simulink model "DQGEN2"  (R2023b)
settings: Solver=ode23tb  StartTime=0.0  StopTime=1  FixedStep=Ts  RelTol=1e-5  EnableMultiTasking=on
values from neighbouring files (symbols this model uses):
  Cd = INVR*SYS.C*Ts    [DQGEN_calc.m]
  N = 2    [DQGEN_calc.m]
  Ts = 50e-6    (= 5e-05)    [DQGEN_calc.m]
  Ts_dqn = Ts    (= 5e-05)    [DQGEN_calc.m]
  Ws = 2*pi*f    (= 376.991118431)    [DQGEN_calc.m]
undefined symbols (not defined in the file or in its folder): ctrl1, Da, DiscIntNeverNeededParam, dtha, FA, Ha, InitVec, Ka, q0, rlc, SM, SMRD, SYS
libraries: spsabctodq0Lib x5, DQN_Lib x5, spsFirstOrderFilterLib x5, spsThreePhaseVIMeasurementLib x3, spsLoadFlowBusLib x2, spsMultimeterLib x2, spsThreePhaseSourceLib x1, spsdq0toabcLib x1, spsGroundLib x1, spsSynchronousMachinepuStandardLib x1, spsThreePhaseParallelRLCBranchLib x1, spsThreePhaseSeriesRLCBranchLib x1
(part 1 of 4)
settings Model: NumberOfSteps=10  PacingRate=0.005000  Creator=The MathWorks, Inc.  LastModifiedBy=rober
settings SolverCC: ZeroCrossControl=DisableAll  ZeroCrossAlgorithm=Adaptive  AlgebraicLoopSolver=TrustRegion
settings DataIOCC: SaveFormat=Array  SaveOutput=off  SaveTime=off  ReturnWorkspaceOutputs=off  TimeSaveName=t  SignalLoggingName=sigsOut
settings OptimizationCC: BlockReduction=off  BooleanDataType=off  ExpressionDepthLimit=2147483647  InitFltsAndDblsToZero=on  EfficientMapNaN2IntZero=off  LifeSpan=inf
settings DebuggingCC: UnderspecifiedInitializationDetection=Classic  MergeDetectMultiDrivingBlocksExec=none  CheckExecutionContextPreStartOutputMsg=on  SignalResolutionControl=TryResolveAllWithWarning  IgnoredZcDiagnostic=none  MultiTaskDSMMsg=warning  MultiTaskCondExecSysMsg=none  FcnCallInpInsideContextMsg=warning  StateNameClashWarn=warning  SFUnexpectedBacktrackingDiag=warning  SFNoUnconditionalDefaultTransitionDiag=warning  SFExecutionAtInitializationDiag=none  UnderSpecifiedDimensionMsg=warning  ArithmeticOperatorsInVariantConditions=warning
settings HardwareCC: ProdBitPerPointer=32  ProdBitPerSizeT=32  ProdBitPerPtrDiffT=32  ProdLargestAtomicFloat=None  ProdIntDivRoundTo=Undefined  ProdEndianess=Unspecified  ProdWordSize=32  ProdHWDeviceType=32-bit Generic  TargetBitPerPointer=64  TargetBitPerSizeT=64  TargetBitPerPtrDiffT=64  TargetLongLongMode=on  TargetIntDivRoundTo=Zero  TargetEndianess=LittleEndian  TargetWordSize=64  TargetHWDeviceType=MATLAB Host  ProdEqTarget=off
settings ModelReferenceCC: EnableRefExpFcnMdlSchedulingChecks=on  PropagateSignalLabelsOutOfModel=off
settings SFSimCC: SimUseLocalCustomCode=off  CustomCodeUndefinedFunction=UseInterfaceOnly
settings RTWCC: RTWUseLocalCustomCode=off  DLArmComputeVersion=19.05
settings CodeAppCC: StateflowObjectComments=on
settings GRTTargetCC: TargetLangStandard=C89/C90 (ANSI)  CombineOutputUpdateFcns=off  GRTInterface=on
settings ConfigComp: CovMetricSettings=dw  CovSaveCumulativeToWorkspaceVar=on  CovSaveSingleToWorkspaceVar=on  CovExternalEMLEnable=off  CovSFcnEnable=off
settings SimscapeCC: SimscapeNormalizeSystem=off

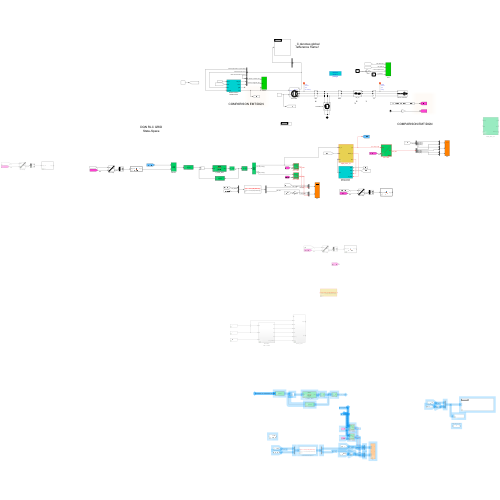
[thumbnail: Simulink's stored preview of the top-level diagram]
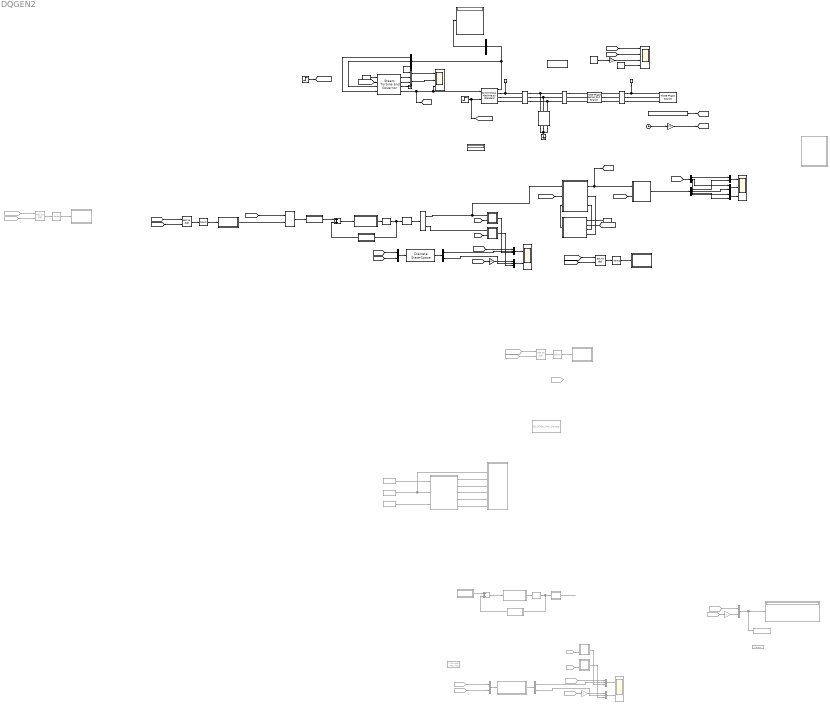
== system DQGEN2 ==
  note: DQN RLC GRID
      | State-Space
  note: 1
  note: 2
  note: 3
  note: 4
  note: COMPARISON EMT/DQN
  note: _C denotes global
      | refference frame!
  note: COMPARISON EMT/DQN
  500 kV 3333 MVA : spsThreePhaseSourceLib/Three-Phase Source  InternalConnection=Yg  VoltagePhases=off  Voltage=(24000)*1  PhaseAngle=0  Voltage_phases=[25e3 25e3 25e3]/sqrt(3)  PhaseAngles_phases=[0 -120 +120]  Frequency=60  NonIdealSource=off  SpecifyImpedance=on  Resistance=3.5  Inductance=0.1989  ShortCircuitLevel=3333e6  BaseVoltage=500e3  XRratio=21.43  BusType=swing  Pref=0  Qref=0  Prefabc=[10e3, 10e3, 10e3]  Qrefabc=[0, 0, 0]  Qmin=-Inf  Qmax=Inf
  Add1 : Sum
  Add2 : Sum  Commented=on
  B1 : spsThreePhaseVIMeasurementLib/Three-Phase V-I Measurement  VoltageMeasurement=phase-to-ground  SetLabelV=on  LabelV=Vabc_BSRC  Vpu=off  VpuLL=off  CurrentMeasurement=yes  SetLabelI=on  LabelI=Iabc_BSRC  Ipu=off  Pbase=100e6  Vbase=500e3  OutputType=Complex  PhasorSimulation=off  PSBequivalent=0
  B22 : spsThreePhaseVIMeasurementLib/Three-Phase V-I Measurement  VoltageMeasurement=phase-to-ground  SetLabelV=on  LabelV=Vabc_B22  Vpu=off  VpuLL=off  CurrentMeasurement=yes  SetLabelI=on  LabelI=Iabc_B222  Ipu=off  Pbase=555e6  Vbase=24e3  OutputType=Complex  PhasorSimulation=off  PSBequivalent=0
  B500 : spsThreePhaseVIMeasurementLib/Three-Phase V-I Measurement  VoltageMeasurement=phase-to-ground  SetLabelV=on  LabelV=Vabc_B500  Vpu=off  VpuLL=off  CurrentMeasurement=yes  SetLabelI=on  LabelI=Iabc_B500  Ipu=off  Pbase=100e6  Vbase=500e3  OutputType=Complex  PhasorSimulation=off  PSBequivalent=0
  Bus Selector1 : BusSelector  OutputSignals="Mechanical.Rotor angle deviation  d_theta (rad),Mechanical.Rotor speed  wm  (pu),Mechanical.Rotor speed deviation  dw (pu)"
  Bus Selector2 : BusSelector  OutputSignals="dq0 components.Stator voltage  vd (pu),dq0 components.Stator voltage  vq (pu),Load angle   delta  (deg)"  OutputAsBus=on
  Clock : Clock
  Constant1 : Constant
  Constant2 : Constant  Value=complex([ 0 (24e3)*sqrt(2/3); 0 0; 0 0])
  Constant3 : Constant  Commented=on  Value=SYS.A
  Constant5 : Constant
  Constant6 : Constant  Commented=on  Value=SYS.B
  Constant7 : Constant  Commented=on  Value=SYS.C
  DQN_Mac1_V1 : Subsystem  mask{HRM=N, NomParam=[ 555e6  24e3   60 ], reactVec=[1.81, 0.3, 0.23, 1.76, 0.65, 0.25, 0.15], timeConstVec=[ 1.3201, 0.0231, 0.3371, 0.0295 ], Rs=2.8544e-3, Mech=[ 0.8788  0 1 ], lfVec=[0.5396   -0.7334    1.0000    1.0315    0.4264], Ts=Ts, SW=on}
      mask prompts: HRM "Harmonic order:"; NomParam "Nominal power, line-to-line voltage, frequency [ Pn(VA)  Vn(Vrms)  fn(Hz) ]:"; reactVec "Reactances [ Xd  Xd'  Xd''  Xq  (Xq')  Xq''  Xl ] (pu):"; timeConstVec "[ Td'  Td''  (Tq')  Tq'' ] (s):"; Rs "Stator resistance Rs (pu):"; Mech "Inertia coefficient, friction factor, pole pairs [ H(s)  F(pu)  p()]:"; lfVec "Initial condition (phi(1x6), tho, dw) [1x8]:"; Ts "Integration timestep (s):"; SW "Method (dq - checked / abc - unchecked)"
      mask init:
      | SMRD = struct();
      | 
      |     SMRD.dwo = 0;
      | 
      |     SMRD.nState = numel(reactVec)-1;
      |     
      |     if(SMRD.nState>5)
      |         SMRD.RLinv   = zeros(6,6);
      |         SMRD.Linv    = zeros(6,6);
      |         SMRD.L       = zeros(6,6);
      |         SMRD.R       = zeros(6,6);
      |         W = zeros(6,6);
      |     else
      |         SMRD.RLinv   = zeros(5,5);
      |         SMRD.Linv    = zeros(5,5);
      |         SMRD.L       = zeros(5,5);
      |         SMRD.R       = zeros(5,5);
      |         W            = zeros(5,5);
      |     end
      | 
      |     SMRD.Rs      = Rs;
      | 
      |     SMRD.N       = 1;
      |     
      |     SMRD.H       = Mech(1);
      |     SMRD.F       = Mech(2);
      |     SMRD.p       = Mech(3);
      | 
      |     SMRD.Pn = NomParam(1);
      |     SMRD.Vn = NomParam(2);
      |     SMRD.fn = NomParam(3);
      |     
      |     
      |     Vb = SMRD.Vn*sqrt(2/3);
      |     Ib = sqrt(2/3)*SMRD.Pn/SMRD.Vn;
      |     
      |     
      |     Td_p    = timeConstVec(1);
      |     Td_pp   = timeConstVec(2);
      |     if(SMRD.nState>5)
      |         Tq_p    = timeConstVec(3);
      |         Tq_pp   = timeConstVec(4);
      |     else
      |         Tq_pp   = timeConstVec(3);
      |     end
      |     
      |     
      |     %Set the time constants in Lq(s)
      |     %See (eq. 7.2.14)
      |     
      |     wn=2*pi*SMRD.fn;
      |     SMRD.wn = wn;%Rated frequency in rad/sec
      |     %Implementation of the formulas in 
      |     
      |     % Xaq=1.165; %Mutual inductance
      |     % Ll=.188; %Stator leakage inductance
      |     
      |     %T5=0.0234;
      |     
      |     
      |     Xd      = reactVec(1);
      |     Xd_p    = reactVec(2);
      |     Xd_pp   = reactVec(3);
      |     Xq      = reactVec(4);
      | 
      | 
      |     if(SMRD.nState>5)
      |         Xq_p    = reactVec(5);
      |         Xq_pp   = reactVec(6);
      |         Xl      = reactVec(7);
      | 
      |         Tqo_p   = Tq_p * Xq/Xq_p;
      |         Tqo_pp  = Tq_pp * Xq_p/Xq_pp;
      |     else
      |         Xq_pp   = reactVec(5);
      |         Xl      = reactVec(6);
      |         Tqo_pp  = Tq_pp * Xq/Xq_pp;
      |     end
      | 
      | 
      |     Xad     = Xd-Xl; %Mutual inductance
      |     Xaq     = Xq-Xl; %Mutual inductance
      |     
      |     
      |     SMRD.Xd = Xd;
      |     SMRD.Xq = Xq;
      |     SMRD.Xl = Xl;
      |     SMRD.Xad = Xad;
      |     SMRD.Xaq = Xaq;
      |     
      |         
      |    
      |     LAM1 = sqrt(Xd^2*Xd_pp^2*(Td_p-Td_pp)^2+2*Td_p*Td_pp*Xd*Xd_p*Xd_pp*(Xd-2*Xd_p+Xd_pp)-2*Td_pp*Xd*Xd_p*Xd_pp*(Xd-Xd_p+Xd_pp)+Td_pp^2*Xd_pp^2*(Xd^2+Xd_pp^2));
      |     Tdo_p  = (Td_p*Xd*Xd_pp+LAM1+Td_pp*(Xd*Xd_p+Xd_p*Xd_pp-Xd*Xd_pp))/(2*Xd_p*Xd_pp);
      |     Tdo_pp = Xd*Td_p*Td_pp/(Xd_pp*Tdo_p);
      |     % 
      |     % Tqo_p   = Tq_p * Xq/Xq_p;
      |     % Tqo_pp  = Tq_pp * Xq_p/Xq_pp;
      | 
      | 
      |     % D-Axis
      |     a=SMRD.Xad*(Xd_p-SMRD.Xl)/(Xd-Xd_p);
      |     b=a*SMRD.Xad*(Xd_pp-SMRD.Xl)/(a*Xd+SMRD.Xl*SMRD.Xad-(a+SMRD.Xad)*Xd_pp);
      |     c=(b+a*SMRD.Xl*SMRD.Xad/(SMRD.Xl*SMRD.Xad+a*Xd))/Td_pp;
      |     
      |     T5 = b/c;
      | 
      |     if(1)
      |         a = Xad*(Xd_p-Xl)/(Xd-Xd_p);
      |         b = Xad*(Xd_pp-Xl)/(a*Xd+Xl*Xad-(a+Xad)*Xd_pp);
      |         c = (1/Td_pp)*(b-(a*Xl*Xad)/(Xl*Xad+a*Xd) );
      |         
      |         T11d = b/c;
      |     end
      | 
      |     
      |     if(1)
      |         %Set the time constants in Ld(s),sG(s)
      |         %See (eq. 7.2.4-7.2.5)
      |         T1 = Td_p; %T1=1.419; %Td'
      |         T2 = Td_pp; %T2=0.0669; %Td''
      |         T3 = Tdo_p; %T3=5.62; %Tdo'
      |         T4 = Tdo_pp; %T4=0.09; %Tdo''
      |         %T5 = T5; %T5=0.0234;
      |         Ld = Xd; %Ld= 1.104; %Synchronous inductance
      |         Ll = Xl; %Ll=0.198; %Stator leakage inductance
      |         Lad = Xad; %Lad=Ld-Ll; %Mutual inductance
      |         %Rated frequency in rad/sec
      |         %Implementation of the formulas in
      | 
      |         T5 = T11d;
      | 
      |         Ro=wn*Ld*(T3+T4-T1-T2);
      |         Ro=Lad*Lad/Ro;
      |         a=Ld*(T1+T2)-Ll*(T3+T4);a=a/Lad;
      |         b=Ld*T1*T2-Ll*T3*T4; b=b/Lad;
      |         c=(T3*T4-T1*T2)/(T3+T4-T1-T2);
      | 
      |         Lf1d=b-a*T5+T5*T5; %in p.u.
      |         Lf1d=Ro*Lf1d/(c-T5); %in p.u.
      |         Rfd=Ro*(Lf1d+Ro*(2*T5-a));
      |         Rfd=Rfd/(Lf1d+Ro*(T5+c-a));%in p.u.
      | 
      |         R1d=Ro*Rfd/(Rfd-Ro); %in p.u.
      |         %Inductances in p.u.
      |         L1d=R1d*T5; 
      |         L1d=L1d*wn;
      | 
      |         Lfd=Rfd*(a-T5-Lf1d/Ro); %in p.u.
      |         Lfd=Lfd*wn; 
      |         Lf1d=Lf1d*wn;
      | 
      |         SMRD.Lf1d = Lf1d;
      |         SMRD.Rfd = Rfd;
      |         SMRD.R1d = R1d;
      |         SMRD.L1d = L1d;
      |         SMRD.Lfd = Lfd;
      |     end
      | 
      | 
      |     %%%%%%%%%%%%%%%%%%%%%%%%% Q AXIS %%%%%%%%%%%%%%%%%%%%%%%%% Tqo′ Xq″ Xq SMRD.Xl 
      |     
      |     if(SMRD.nState>5)
      |         %conv(x,y)= polynomial multiplication
      |         N=conv([Tq_p 1],[Tq_pp 1]); 
      |         D=conv([Tqo_p 1],[Tqo_pp 1]);
      |         Nz=conv(N-D*SMRD.Xl/Xq,[Xaq/SMRD.wn 0]);
      |         Dz=D-N; Nz=Nz(1:3); Dz=Dz(1:2);
      |         Req=Nz(3)/Dz(2);
      |         Nz=Nz/Nz(3); Dz=Dz/Dz(2);
      |         %compute polynomial roots and sort them
      |         Tab=sort(abs(roots(Nz))); Tab=1./Tab;
      |         Tm=sort(abs(roots(Dz))); Tm=1/Tm(1);
      |         %Solve a system of two linear equa�tions
      |         x=[1 1;Tab(1) Tab(2)]\[1 ;Tm]/Req;
      |         %Results
      |         SMRD.R1q=1/x(1); 
      |         SMRD.L1q=SMRD.wn*SMRD.R1q*Tab(1); %in p.u.
      |         SMRD.R2q=1/x(2); 
      |         SMRD.L2q=SMRD.wn*SMRD.R2q*Tab(2); %in p.u.
      |     else
      |         N=conv([1],[Tq_pp 1]); 
      |         D=conv([1],[Tqo_pp 1]);
      |         Nz=conv(N-D*SMRD.Xl/Xq,[Xaq/SMRD.wn 0]);
      |         Dz=D-N; Nz=Nz(1:2); Dz=Dz(1:1);
      |         Req=Nz(2)/Dz(1);
      |         Nz=Nz/Nz(2); Dz=Dz/Dz(1);
      |         %compute polynomial roots and sort them
      |         Tab=sort(abs(roots(Nz))); Tab=1./Tab;
      |         Tm=1;
      |         %Solve a system of two linear equa�tions
      |         x=[1;Tab(1)]/Req;
      |         %Results
      |         SMRD.R1q=1/x(1); 
      |         SMRD.L1q=SMRD.wn*SMRD.R1q*Tab(1); %in p.u.
      |     end
      |     
      |     %%%%%%%%%%%%%%%%%%%%%%%%%%%%%%%%%%%%%%%%%%%%%%%%%%%%%%%%%%
      | 
      |     %%%%%%%%%%%%%%%%%%%%%%%%% R/L MAT %%%%%%%%%%%%%%%%%%%%%%%%%
      | 
      |     q_axis = 1;
      | 
      | 
      |     if(SMRD.nState>5) % D = 2,3,4 ; Q = 1,5,6
      | 
      |         if(q_axis)
      |             SMRD.L(2,2) = SMRD.Xd;  SMRD.L(2,3) = SMRD.Xad;                         SMRD.L(2,4) = SMRD.Xad; %D
      |             SMRD.L(3,2) = SMRD.Xad; SMRD.L(3,3) = SMRD.Xad + SMRD.Lf1d + SMRD.Lfd;  SMRD.L(3,4) = SMRD.Lf1d + SMRD.Xad; %D
      |             SMRD.L(4,2) = SMRD.Xad; SMRD.L(4,3) = SMRD.Xad + SMRD.Lf1d;             SMRD.L(4,4) = SMRD.Lf1d + SMRD.Xad + SMRD.L1d; %D
      | 
      |             SMRD.L(1,1) = SMRD.Xq;  SMRD.L(1,5) = SMRD.Xaq;                         SMRD.L(1,6) = SMRD.Xaq; %Q
      |             SMRD.L(5,1) = SMRD.Xaq; SMRD.L(5,5) = SMRD.Xaq + SMRD.L1q;              SMRD.L(5,6) = SMRD.Xaq; %Q
      |             SMRD.L(6,1) = SMRD.Xaq; SMRD.L(6,5) = SMRD.Xaq;                         SMRD.L(6,6) = SMRD.Xaq + SMRD.L2q; %Q
      | 
      | 
      |             SMRD.R(1,1) = Rs;
      |             SMRD.R(2,2) = Rs;
      |             SMRD.R(3,3) = SMRD.Rfd;
      |             SMRD.R(4,4) = SMRD.R1d;
      |             SMRD.R(5,5) = SMRD.R1q;
      |             SMRD.R(6,6) = SMRD.R2q;
      | 
      |         else
      |             SMRD.L(1,1) = SMRD.Xd;  SMRD.L(1,3) = SMRD.Xad;                         SMRD.L(1,5) = SMRD.Xad;
      |             SMRD.L(2,2) = SMRD.Xq;  SMRD.L(2,4) = SMRD.Xaq;                         SMRD.L(2,6) = SMRD.Xaq;
      |             SMRD.L(3,1) = SMRD.Xad; SMRD.L(3,3) = SMRD.Xad + SMRD.Lf1d + SMRD.Lfd;  SMRD.L(3,5) = SMRD.Lf1d + SMRD.Xad;
      |             SMRD.L(4,2) = SMRD.Xaq; SMRD.L(4,4) = SMRD.Xaq + SMRD.L1q;              SMRD.L(4,6) = SMRD.Xaq;
      |             SMRD.L(5,1) = SMRD.Xad; SMRD.L(5,3) = SMRD.Xad + SMRD.Lf1d;             SMRD.L(5,5) = SMRD.Lf1d + SMRD.Xad + SMRD.L1d;
      |             SMRD.L(6,2) = SMRD.Xaq; SMRD.L(6,4) = SMRD.Xaq;                         SMRD.L(6,6) = SMRD.Xaq  + SMRD.L2q;
      | 
      |             SMRD.R(1,1) = Rs;
      |             SMRD.R(2,2) = Rs;
      |             SMRD.R(3,3) = SMRD.Rfd;
      |             SMRD.R(4,4) = SMRD.R1q;
      |             SMRD.R(5,5) = SMRD.R1d;
      |             SMRD.R(6,6) = SMRD.R2q;
      |         end
      |     else
      | 
      |         if(q_axis)
      |             SMRD.L(2,2) = SMRD.Xd;  SMRD.L(2,3) = SMRD.Xad;                         SMRD.L(2,4) = SMRD.Xad;           %D
      |             SMRD.L(3,2) = SMRD.Xad; SMRD.L(3,3) = SMRD.Xad + SMRD.Lf1d + SMRD.Lfd;  SMRD.L(3,4) = SMRD.Lf1d + SMRD.Xad; %D
      |             SMRD.L(4,2) = SMRD.Xad; SMRD.L(4,3) = SMRD.Xad + SMRD.Lf1d;             SMRD.L(4,4) = SMRD.Lf1d + SMRD.Xad + SMRD.L1d;  %D
      |             
      |             SMRD.L(1,1) = SMRD.Xq;  SMRD.L(1,5) = SMRD.Xaq;              %Q
      |             SMRD.L(5,1) = SMRD.Xaq; SMRD.L(5,5) = SMRD.Xaq + SMRD.L1q;   %Q
      | 
      |             SMRD.R(1,1) = Rs;
      |             SMRD.R(2,2) = Rs;
      |             SMRD.R(3,3) = Rfd_R;
      |             SMRD.R(4,4) = R1d_R;
      |             SMRD.R(5,5) = SMRD.R1q;
      | 
      |         else
      |             SMRD.L(1,1) = SMRD.Xd; SMRD.L(1,3) = SMRD.Xad; SMRD.L(1,5) = SMRD.Xad;
      |             SMRD.L(2,2) = SMRD.Xq; SMRD.L(2,4) = SMRD.Xaq;
      |             SMRD.L(3,1) = SMRD.Xad; SMRD.L(3,3) = SMRD.Xad + SMRD.Lf1d + SMRD.L1d; SMRD.L(3,5) = SMRD.Lf1d + SMRD.Xad;
      |             SMRD.L(4,2) = SMRD.Xaq; SMRD.L(4,4) = SMRD.Xaq + SMRD.L1q; 
      |             SMRD.L(5,1) = SMRD.Xad; SMRD.L(5,3) = SMRD.Xad + SMRD.Lf1d; SMRD.L(5,5) = SMRD.Lf1d + SMRD.Xad + SMRD.Lfd;
      | 
      |             SMRD.R(1,1) = Rs;
      |             SMRD.R(2,2) = Rs;
      |             SMRD.R(3,3) = Rfd_R;
      |             SMRD.R(4,4) = SMRD.R1q;
      |             SMRD.R(5,5) = R1d_R;
      | 
      |         end
      |     end
      | 
      | 
      |    if(q_axis)
      |         W(2,1) = -1;
      |         W(1,2) = +1;
      |    else
      |         W(2,1) = +1;
      |         W(1,2) = -1;
      |    end
      |     
      |     %%%%%%%%%%%%%%%%%%%%%%%%%%%%% LF  %%%%%%%%%%%%%%%%%%%%%%%%%
      |     
      |     Pt = lfVec(1);
      |     Qt = lfVec(2);
      |     Vt = lfVec(3);
      |     Et = lfVec(4);
      |     At = lfVec(5);
      |     % if(numel(lfVec)>5) fac = lfVec(6); end
      |     
      |     phi = At;
      |     SMRD.phi = phi;
      | 
      |     SMRD.Vt = Vt*exp(1i*(phi));
      |     SMRD.It = (Pt-1i*Qt)/(Vt*exp(-1i*(phi)));
      |        
      |     %fi = sign(Qt)*acos(Pt/(Vt*It)); rad2deg(fi);
      |     fi = angle(SMRD.Vt)-angle(SMRD.It);
      |     SMRD.fi = fi;
      |     
      |     % del = (atan((Xq*It*cos(fi)-Rs*It*sin(fi))/(Vt+Rs*It*cos(fi)+Xq*It*sin(fi))));
      |     del = angle(SMRD.Vt+(SMRD.Rs+1i*SMRD.Xq)*SMRD.It)-(SMRD.phi);
      | 
      |     SMRD.del = del;
      | 
      |     SMRD.Vfnp = ((SMRD.Rfd*Vb/(Xad*wn))^2);
      |     
      |     v_dq = Vt*exp(1i*(pi/2-del)); %correct
      |     ed = real(v_dq);
      |     eq = imag(v_dq);
      |     efd = Et*SMRD.Vfnp;
      |     
      |    if(q_axis)
      |         v_vec = [eq; ed; efd; zeros(SMRD.nState-3,1)];
      |         i_vec = (v_vec'/(SMRD.R-SMRD.L*W))';
      |    else
      |         v_vec = [ed; eq; efd; zeros(SMRD.nState-3,1)];
      |         i_vec = (v_vec'/(SMRD.R-SMRD.L*W))';
      |    end
      | 
      |     %%%%%%%%%%%%%%%%%%%%%%%%%%%%%%%%%%%%%%%%%%%%%%%%%%%%%%%%%%
      |     
      |     SMRD.idq0 = i_vec;
      |     SMRD.phidq0 = SMRD.L*i_vec;
      |     
      |     SMRD.dwo = 0;
      | 
      |     SMRD.Linv = eye(SMRD.nState)/SMRD.L;
      |     
      |     if(1)
      |         SMRD.Linv2 = SMRD.Linv;
      |         SMRD.Linv2(3,4) = 0; SMRD.Linv2(4,3) = 0;
      |     end
      | 
      | 
      |     SMRD.RLinv = SMRD.R*SMRD.Linv;
      | 
      | 
      |     SMRD.Pb = 1;
      |     SMRD.Ib = Ib;
      |     SMRD.Vb = Vb;
      | 
      |     SMRD.IqdSign = [-1    -1     ones(1,SMRD.nState-2)];
      | 
      | 
      |     SMRD.Ts = Ts;
      |     SMRD.web = SMRD.wn;
      |     SMRD.v_dq = v_dq;
      | 
      |     tho = del+phi-pi/2;
      |     SMRD.tho = tho;
      settings: LibrarySourceBlock=|
      | spsSynchronousMachineModel/Continuous/Synchronous Machine
      | Continuous Model
  DQN_Mac_V1 : Subsystem  Commented=on  mask{HRM=N, NomParam=[ 555e6  24e3   60 ], reactVec=[1.81, 0.3, 0.23, 1.76, 0.65, 0.25, 0.15], timeConstVec=[ 1.3201, 0.0231, 0.3371, 0.0295 ], Rs=3.10E-03, Mech=[ 0.8788  0 1 ], lfVec=[0.9000   -0.0895    1.0000    1.8333    0.3334], Ts=Ts}
      mask prompts: HRM "Harmonic order:"; NomParam "Nominal power, line-to-line voltage, frequency [ Pn(VA)  Vn(Vrms)  fn(Hz) ]:"; reactVec "Reactances [ Xd  Xd'  Xd''  Xq  (Xq')  Xq''  Xl ] (pu):"; timeConstVec "[ Td'  Td''  (Tq')  Tq'' ] (s):"; Rs "Stator resistance Rs (pu):"; Mech "Inertia coefficient, friction factor, pole pairs [ H(s)  F(pu)  p()]:"; lfVec "Initial condition (phi(1x6), tho, dw) [1x8]:"; Ts "Integration timestep (s):"
      mask init:
      | SMRD = struct();
      | 
      |     SMRD.dwo = 0;
      | 
      |     SMRD.nState = numel(reactVec)-1;
      |     
      |     if(SMRD.nState>5)
      |         SMRD.RLinv   = zeros(6,6);
      |         SMRD.Linv    = zeros(6,6);
      |         SMRD.L       = zeros(6,6);
      |         SMRD.R       = zeros(6,6);
      |         W = zeros(6,6);
      |     else
      |         SMRD.RLinv   = zeros(5,5);
      |         SMRD.Linv    = zeros(5,5);
      |         SMRD.L       = zeros(5,5);
      |         SMRD.R       = zeros(5,5);
      |         W            = zeros(5,5);
      |     end
      | 
      |     SMRD.Rs      = Rs;
      | 
      |     SMRD.N       = 1;
      |     
      |     SMRD.H       = Mech(1);
      |     SMRD.F       = Mech(2);
      |     SMRD.p       = Mech(3);
      | 
      |     SMRD.Pn = NomParam(1);
      |     SMRD.Vn = NomParam(2);
      |     SMRD.fn = NomParam(3);
      |     
      |     
      |     Vb = SMRD.Vn*sqrt(2/3);
      |     Ib = sqrt(2/3)*SMRD.Pn/SMRD.Vn;
      |     
      |     
      |     Td_p    = timeConstVec(1);
      |     Td_pp   = timeConstVec(2);
      |     if(SMRD.nState>5)
      |         Tq_p    = timeConstVec(3);
      |         Tq_pp   = timeConstVec(4);
      |     else
      |         Tq_pp   = timeConstVec(3);
      |     end
      |     
      |     
      |     %Set the time constants in Lq(s)
      |     %See (eq. 7.2.14)
      |     
      |     wn=2*pi*SMRD.fn;
      |     SMRD.wn = wn;%Rated frequency in rad/sec
      |     %Implementation of the formulas in 
      |     
      |     % Xaq=1.165; %Mutual inductance
      |     % Ll=.188; %Stator leakage inductance
      |     
      |     %T5=0.0234;
      |     
      |     
      |     Xd      = reactVec(1);
      |     Xd_p    = reactVec(2);
      |     Xd_pp   = reactVec(3);
      |     Xq      = reactVec(4);
      | 
      | 
      |     if(SMRD.nState>5)
      |         Xq_p    = reactVec(5);
      |         Xq_pp   = reactVec(6);
      |         Xl      = reactVec(7);
      | 
      |         Tqo_p   = Tq_p * Xq/Xq_p;
      |         Tqo_pp  = Tq_pp * Xq_p/Xq_pp;
      |     else
      |         Xq_pp   = reactVec(5);
      |         Xl      = reactVec(6);
      |         Tqo_pp  = Tq_pp * Xq/Xq_pp;
      |     end
      | 
      | 
      |     Xad     = Xd-Xl; %Mutual inductance
      |     Xaq     = Xq-Xl; %Mutual inductance
      |     
      |     
      |     SMRD.Xd = Xd;
      |     SMRD.Xq = Xq;
      |     SMRD.Xl = Xl;
      |     SMRD.Xad = Xad;
      |     SMRD.Xaq = Xaq;
      |     
      |         
      |    
      |     LAM1 = sqrt(Xd^2*Xd_pp^2*(Td_p-Td_pp)^2+2*Td_p*Td_pp*Xd*Xd_p*Xd_pp*(Xd-2*Xd_p+Xd_pp)-2*Td_pp*Xd*Xd_p*Xd_pp*(Xd-Xd_p+Xd_pp)+Td_pp^2*Xd_pp^2*(Xd^2+Xd_pp^2));
      |     Tdo_p  = (Td_p*Xd*Xd_pp+LAM1+Td_pp*(Xd*Xd_p+Xd_p*Xd_pp-Xd*Xd_pp))/(2*Xd_p*Xd_pp);
      |     Tdo_pp = Xd*Td_p*Td_pp/(Xd_pp*Tdo_p);
      |     % 
      |     % Tqo_p   = Tq_p * Xq/Xq_p;
      |     % Tqo_pp  = Tq_pp * Xq_p/Xq_pp;
      |     
      |    
      |     %%%%%%%%%%%%%%%%%%%%%%
      |         
      |     a=SMRD.Xad*(Xd_p-SMRD.Xl)/(Xd-Xd_p);
      |     b=a*SMRD.Xad*(Xd_pp-SMRD.Xl)/(a*Xd+SMRD.Xl*SMRD.Xad-(a+SMRD.Xad)*Xd_pp);
      |     c=(b+a*SMRD.Xl*SMRD.Xad/(SMRD.Xl*SMRD.Xad+a*Xd))/Td_pp;
      |     
      |     T5 = b/c;
      |     
      |     %%%%%%%%%%%%%%%%%%%%%%%%% D AXIS %%%%%%%%%%%%%%%%%%%%%%%%%
      |     
      |     SMRD.Ro=SMRD.wn*Xd*(Tdo_p+Tdo_pp-Td_p-Td_pp);
      |     SMRD.Ro=SMRD.Xad*SMRD.Xad/SMRD.Ro;
      |     
      |     
      |     a=Xd*(Td_p+Td_pp)-SMRD.Xl*(Tdo_p+Tdo_pp);a=a/SMRD.Xad;
      |     b=Xd*Td_p*Td_pp-SMRD.Xl*Tdo_p*Tdo_pp; b=b/SMRD.Xad;
      |     c=(Tdo_p*Tdo_pp-Td_p*Td_pp)/(Tdo_p+Tdo_pp-Td_p-Td_pp);
      |     
      |     % T5=0.0234;
      |     
      |     SMRD.Lf1d=b-a*T5+T5*T5; %in p.u.
      |     SMRD.Lf1d=SMRD.Ro*SMRD.Lf1d/(c-T5); %in p.u.
      |     SMRD.Rfd=SMRD.Ro*(SMRD.Lf1d+SMRD.Ro*(2*T5-a)); 
      |     SMRD.Rfd=SMRD.Rfd/(SMRD.Lf1d+SMRD.Ro*(T5+c-a));%in p.u.
      |     SMRD.Lfd=SMRD.Rfd*(a-T5-SMRD.Lf1d/SMRD.Ro); %in p.u.
      |     SMRD.R1d=SMRD.Ro*SMRD.Rfd/(SMRD.Rfd-SMRD.Ro); %in p.u. 
      |     %Inductances in p.u.
      |     SMRD.L1d=SMRD.R1d*T5; SMRD.L1d=SMRD.L1d*SMRD.wn; 
      |     SMRD.Lfd=SMRD.Lfd*SMRD.wn; SMRD.Lf1d=SMRD.Lf1d*SMRD.wn;
      |     
      |     %%%%%%%%%%%%%%%%%%%%%%%%%%%%%%%%%%%%%%%%%%%%%%%%%%%%%%%%%%
      |     
      |     %%%%%%%%%%%%%%%%%%%%%%%%% Q AXIS %%%%%%%%%%%%%%%%%%%%%%%%% Tqo′ Xq″ Xq SMRD.Xl 
      |     
      |     if(SMRD.nState>5)
      |         %conv(x,y)= polynomial multiplication
      |         N=conv([Tq_p 1],[Tq_pp 1]); 
      |         D=conv([Tqo_p 1],[Tqo_pp 1]);
      |         Nz=conv(N-D*SMRD.Xl/Xq,[Xaq/SMRD.wn 0]);
      |         Dz=D-N; Nz=Nz(1:3); Dz=Dz(1:2);
      |         Req=Nz(3)/Dz(2);
      |         Nz=Nz/Nz(3); Dz=Dz/Dz(2);
      |         %compute polynomial roots and sort them
      |         Tab=sort(abs(roots(Nz))); Tab=1./Tab;
      |         Tm=sort(abs(roots(Dz))); Tm=1/Tm(1);
      |         %Solve a system of two linear equa�tions
      |         x=[1 1;Tab(1) Tab(2)]\[1 ;Tm]/Req;
      |         %Results
      |         SMRD.R1q=1/x(1); 
      |         SMRD.L1q=SMRD.wn*SMRD.R1q*Tab(1); %in p.u.
      |         SMRD.R2q=1/x(2); 
      |         SMRD.L2q=SMRD.wn*SMRD.R2q*Tab(2); %in p.u.
      |     else
      |         N=conv([1],[Tq_pp 1]); 
      |         D=conv([1],[Tqo_pp 1]);
      |         Nz=conv(N-D*SMRD.Xl/Xq,[Xaq/SMRD.wn 0]);
      |         Dz=D-N; Nz=Nz(1:2); Dz=Dz(1:1);
      |         Req=Nz(2)/Dz(1);
      |         Nz=Nz/Nz(2); Dz=Dz/Dz(1);
      |         %compute polynomial roots and sort them
      |         Tab=sort(abs(roots(Nz))); Tab=1./Tab;
      |         Tm=1;
      |         %Solve a system of two linear equa�tions
      |         x=[1;Tab(1)]/Req;
      |         %Results
      |         SMRD.R1q=1/x(1); 
      |         SMRD.L1q=SMRD.wn*SMRD.R1q*Tab(1); %in p.u.
      |     end
      |     
      |     %%%%%%%%%%%%%%%%%%%%%%%%%%%%%%%%%%%%%%%%%%%%%%%%%%%%%%%%%%
      |     
      |     
      |     if(1)
      |         T11d = T5;
      |         
      |         K1 = (Tdo_p+Tdo_pp-Td_p-Td_pp)*(Tdo_p*Tdo_pp*(Td_p+Td_pp)-Td_p*Td_pp*(Tdo_p+Tdo_pp))-(Tdo_p*Tdo_pp-Td_p*Td_pp)^2;    
      |         
      |         
      |         %K2 = Rfd*K1*Ld/(Lad^2);
      |         K2 = (Tdo_p*Tdo_pp*(Td_p+Td_pp)-Td_p*Td_pp*(Tdo_p+Tdo_pp)+T11d^2*(Tdo_p+Tdo_pp-Td_p-Td_pp)-2*T11d*(Tdo_p*Tdo_pp-Td_p*Td_pp))/SMRD.wn;
      |         K3 = Tdo_p*Tdo_pp-T11d*(Tdo_p+Tdo_pp-T11d);
      |         K4 = Tdo_p*Tdo_pp-Td_p*Td_pp-T11d*(Tdo_p+Tdo_pp-Td_p-Td_pp);
      |         K5 = Tdo_p*Tdo_pp*(Td_p+Td_pp)-Td_p*Td_pp*(Tdo_p+Tdo_pp)-T11d*(Tdo_p*Tdo_pp-Td_p*Td_pp);
      |         
      |         Rfd_R = Xad^2*K2/(Xd*K1);
      |         
      |         Lf1d_R = (Xad^2*K3/(Xd*K4)-Xad)*wn; %Lf1d
      |         Lfd_R = Rfd_R*K5/K4*wn; %Lfd
      |         R1d_R = Rfd_R*K1/K4^2;
      |         L1d_R = Rfd_R*T5*wn;
      |         
      |         SMRD.Rfd_R  = Rfd_R;
      |         SMRD.Lf1d_R = Lf1d_R;
      |         SMRD.Lfd_R = Lfd_R;
      |         SMRD.R1d_R = R1d_R;
      |         SMRD.L1d_R = L1d_R;
      |     end
      |     
      | 
      |     %%%%%%%%%%%%%%%%%%%%%%%%% R/L MAT %%%%%%%%%%%%%%%%%%%%%%%%%
      | 
      |     Ro=Xad*Xad/(wn*Xd*(Tdo_p+Tdo_pp-Td_p-Td_pp));
      | 
      |     if(SMRD.nState>5)
      |         SMRD.L(1,1) = SMRD.Xd; SMRD.L(1,3) = SMRD.Xad; SMRD.L(1,5) = SMRD.Xad;
      |         SMRD.L(2,2) = SMRD.Xq; SMRD.L(2,4) = SMRD.Xaq; SMRD.L(2,6) = SMRD.Xaq;
      |         SMRD.L(3,1) = SMRD.Xad; SMRD.L(3,3) = SMRD.Xad + SMRD.Lf1d + SMRD.L1d; SMRD.L(3,5) = SMRD.Lf1d + SMRD.Xad;
      |         SMRD.L(4,2) = SMRD.Xaq; SMRD.L(4,4) = SMRD.Xaq + SMRD.L1q; SMRD.L(4,6) = SMRD.Xaq;
      |         SMRD.L(5,1) = SMRD.Xad; SMRD.L(5,3) = SMRD.Xad + SMRD.Lf1d; SMRD.L(5,5) = SMRD.Lf1d + SMRD.Xad + SMRD.Lfd;
      |         SMRD.L(6,2) = SMRD.Xaq; SMRD.L(6,4) = SMRD.Xaq; SMRD.L(6,6) = SMRD.Xaq + SMRD.L2q;
      |     else
      |         SMRD.L(1,1) = SMRD.Xd; SMRD.L(1,3) = SMRD.Xad; SMRD.L(1,5) = SMRD.Xad;
      |         SMRD.L(2,2) = SMRD.Xq; SMRD.L(2,4) = SMRD.Xaq; %SMRD.L(2,6) = SMRD.Xaq;
      |         SMRD.L(3,1) = SMRD.Xad; SMRD.L(3,3) = SMRD.Xad + SMRD.Lf1d + SMRD.L1d; SMRD.L(3,5) = SMRD.Lf1d + SMRD.Xad;
      |         SMRD.L(4,2) = SMRD.Xaq; SMRD.L(4,4) = SMRD.Xaq + SMRD.L1q; %SMRD.L(4,6) = SMRD.Xaq;
      |         SMRD.L(5,1) = SMRD.Xad; SMRD.L(5,3) = SMRD.Xad + SMRD.Lf1d; SMRD.L(5,5) = SMRD.Lf1d + SMRD.Xad + SMRD.Lfd;
      |         %SMRD.L(6,2) = SMRD.Xaq; SMRD.L(6,4) = SMRD.Xaq; SMRD.L(6,6) = SMRD.Xaq + SMRD.L2q;
      |     end
      |     
      |     
      | 
      |     
      |     W(2,1) = +1;
      |     W(1,2) = -1;
      |     
      |    if(SMRD.nState>5) 
      |     SMRD.R(1,1) = Rs;
      |     SMRD.R(2,2) = Rs;
      |     SMRD.R(3,3) = Rfd_R;
      |     SMRD.R(4,4) = SMRD.R1q;
      |     SMRD.R(5,5) = R1d_R;
      |     SMRD.R(6,6) = SMRD.R2q;
      |    else
      |     SMRD.R(1,1) = Rs;
      |     SMRD.R(2,2) = Rs;
      |     SMRD.R(3,3) = Rfd_R;
      |     SMRD.R(4,4) = SMRD.R1q;
      |     SMRD.R(5,5) = R1d_R;
      |    end
      |     
      |     %%%%%%%%%%%%%%%%%%%%%%%%%%%%%%%%%%%%%%%%%%%%%%%%%%%%%%%%%%
      |     
      |     
      |     a=(Xd*(Td_p+Td_pp)-Xl*(Tdo_p+Tdo_pp))/Xad;
      |     b=(Xd*Td_p*Td_pp-Xl*Tdo_p*Tdo_pp)/Xad;
      |     c=(Tdo_p*Tdo_pp-Td_p*Td_pp)/(Tdo_p+Tdo_pp-Td_p-Td_pp);
      |     Lf1d=b-a*T5+T5*T5; %in p.u.
      |     Lf1d=Ro*Lf1d/(c-T5); %in p.u.
      |     %Rfd=Ro*(Lf1d+Ro*(2*T5-a));
      |     Rfd=Ro*(Lf1d+Ro*(2*T5-a))/(Lf1d+Ro*(T5+c-a));%in p.u.
      |     Lfd=Rfd*(a-T5-Lf1d/Ro); %in p.u.
      |     R1d=Ro*Rfd/(Rfd-Ro); %in p.u.
      |     %Inductances in p.u.
      |     L1d=R1d*T5; 
      |     L1d=L1d*wn;
      |     Lfd=Lfd*wn; 
      |     Lf1d=Lf1d*wn;
      |      
      |     
      |     a = Xad*(Xd_p-Xl)/(Xd-Xd_p);
      |     b = Xad*(Xd_pp-Xl)/(a*Xd+Xl*Xad-(a+Xad)*Xd_pp);
      |     c = (1/Td_pp)*(b- (a*Xl*Xad)/(Xl*Xad+a*Xd) );
      |     
      |     T11d = b/c;
      |     
      |     
      |     Xf1d = Xad^2*K3/(Xd*K4)-Xad;
      |     X1d = T11d*Rfd - K1/K4^2;
      |     
      |     SMRD.Xf1d = Xf1d;
      |     SMRD.X1d = X1d;
      |     
      |     %%%%%%%%%%%%%%%%%%%%%%%%%%%%% LF  %%%%%%%%%%%%%%%%%%%%%%%%%
      |     
      |     Pt = lfVec(1);
      |     Qt = lfVec(2);
      |     Vt = lfVec(3);
      |     Et = lfVec(4);
      |     At = lfVec(5);
      |     % if(numel(lfVec)>5) fac = lfVec(6); end
      |     
      |     phi = At;
      |     
      |     It = sqrt(Pt^2+Qt^2)/Vt; 
      |     
      |     Xd = reactVec(1);
      |     Xq = reactVec(4);
      | 
      |     Xmd = Xd-Xl;
      |     
      |     fi = sign(Qt)*acos(Pt/(Vt*It)); rad2deg(fi)
      |     
      |     del = (atan((Xq*It*cos(fi)-Rs*It*sin(fi))/(Vt+Rs*It*cos(fi)+Xq*It*sin(fi))));
      |     
      |     SMRD.del = del;
      |     
      |     tho = del+phi-pi/2;
      |     
      |     SMRD.Vfnp = ((Rfd*Vb/(Xmd*wn))^2);
      |     
      |     v_dq = Vt*exp(1i*(pi/2-del)); %correct
      |     ed = real(v_dq);
      |     eq = imag(v_dq);
      |     efd = Et*SMRD.Vfnp;
      |     
      |     
      |     v_vec = [ed; eq; efd; zeros(SMRD.nState-3,1)];
      |     i_vec = (v_vec'/(SMRD.R-SMRD.L*W))';
      | 
      |     %%%%%%%%%%%%%%%%%%%%%%%%%%%%%%%%%%%%%%%%%%%%%%%%%%%%%%%%%%
      |     
      |     SMRD.idq0 = i_vec;
      |     SMRD.phidq0 = SMRD.L*i_vec;
      |     SMRD.tho = tho;
      |     SMRD.dwo = 0;
      | 
      |     SMRD.Linv = eye(SMRD.nState)/SMRD.L;
      |     SMRD.RLinv = SMRD.R*SMRD.Linv;
      | 
      | 
      |     SMRD.Pb = 1;
      |     SMRD.Ib = Ib;
      |     SMRD.Vb = Vb;
      | 
      |     SMRD.IqdSign = [-1    -1     ones(1,SMRD.nState-2)];
      | 
      |     SMRD.Vt = Vt*exp(1i*(phi));
      |     SMRD.It = (Pt-1i*Qt)/(Vt*exp(-1i*(phi)));
      |     SMRD.Ts = Ts;
      |     SMRD.web = SMRD.wn;
      settings: LibrarySourceBlock=|
      | spsSynchronousMachineModel/Continuous/Synchronous Machine
      | Continuous Model
  DQn->ABC : MATLAB Function  TreatAsAtomicUnit=on  SystemSampleTime=Ts  mask{N=N}
      mask prompts: N "Harmonic order:"
  DQn->ABC1 : MATLAB Function  TreatAsAtomicUnit=on  SystemSampleTime=Ts  mask{N=N}
      mask prompts: N "Harmonic order:"
  DQn->ABC2 : MATLAB Function  TreatAsAtomicUnit=on  SystemSampleTime=Ts  mask{N=N}
      mask prompts: N "Harmonic order:"
  DQn->ABC3 : MATLAB Function  Commented=on  TreatAsAtomicUnit=on  SystemSampleTime=Ts  mask{N=N}
      mask prompts: N "Harmonic order:"
  DQn->ABC4 : MATLAB Function  Commented=on  TreatAsAtomicUnit=on  SystemSampleTime=Ts  mask{N=N}
      mask prompts: N "Harmonic order:"
  Demux : Demux  Outputs=2
  Demux1 : Demux  Commented=on  Outputs=2
  Demux6 : Demux  Outputs=3
  Demux7 : Demux  Outputs=3
  Demux_DQNc_Mat2 : DQN_Lib/Demux_DQNc_Mat  nrOut=2
  Discrete State-Space : DQN_Lib/Discrete State-Space  A=SYS.A  B=SYS.B  C=SYS.C  D=SYS.D  InitVec=SYS.x0  dt=Ts
      settings: LibrarySourceBlock=|
      | spsSynchronousMachineModel/Discrete robust/State Space Model/Discretize
      | BE or Tustin
  Discrete State-Space1 : Subsystem  Commented=on  mask{A=SYS.A, B=SYS.B, C=SYS.C, D=SYS.D, InitVec=InitVec', dt=Ts}
      mask prompts: InitVec "Initial condition:"; dt "Time step (s):"
      mask init:
      | I = eye(size(A,1));
      | INVR = I/(I-A*dt/2);
      | Ad1 = INVR*(I+A*dt/2);
      | Bd1 = INVR*B*dt/2;
      | Cd1 = C*Ad1;
      | Cd = INVR*C*dt;
      | Dd11 = C*INVR*B*dt/2+D;
      | Dd12 = C*INVR*B*dt/2;
      settings: LibrarySourceBlock=|
      | spsSynchronousMachineModel/Discrete robust/State Space Model/Discretize
      | BE or Tustin
      mask Display: disp(['{\color{red}\bf\fontsize{12}x(t) = Ad*x(t-dt)+Bd*u(t)}',newline,'{\color{gray}\bf\fontsize{12}y(t) = Cd*x(t-dt)+Dd*u(t)}'], 'texmode','on');
  Discretize BE or Tustin : Subsystem  Commented=on  AncestorBlock="DQN_Machines/DQN_Mac_V1/Discretize  BE or Tustin"
  Display : Display
  Display1 : Display
  Display2 : Display  Commented=on
  From{5,12,20,22} (4 alike) : From  Commented=on  GotoTag=theta0
  From17 : From  Commented=on  GotoTag=VSRC_C
  From18 : From  Commented=on  GotoTag=Iabc_B222  TagVisibility=global
  From21 : From  Commented=on  GotoTag=Vabc_BSRC  TagVisibility=global
  From23 : From  Commented=on  GotoTag=Vabc_B22  TagVisibility=global
  From24 : From  Commented=on  GotoTag=Iabc_B500  TagVisibility=global
  From25 : From  Commented=on  GotoTag=Iabc_B222  TagVisibility=global
  From26 : From  Commented=on  GotoTag=Iabc_B500  TagVisibility=global
  From27 : From  Commented=on  GotoTag=Vabc_B22  TagVisibility=global
  From6 : From  Commented=on  GotoTag=Vabc_B22  TagVisibility=global
  Gain1 : Gain  Gain=-1
  Gain12 : Gain  Gain=Ws
  Gain2 : Gain  Commented=on  Gain=-1
  Gain3 : Gain  Commented=on  Gain=-1
  Gain_DQNc_Mat1 : MATLAB Function  TreatAsAtomicUnit=on  SystemSampleTime=Ts  mask{Rabc=SYS.C, HRM=N, chkInv=off}
      mask prompts: Rabc "Line matrix [3x3]:"; HRM "Harmonic order:"; chkInv "Invert"
  Gain_DQNc_Mat2 : MATLAB Function  TreatAsAtomicUnit=on  SystemSampleTime=Ts  mask{Rabc=SYS.A, HRM=N, chkInv=off}
      mask prompts: Rabc "Line matrix [3x3]:"; HRM "Harmonic order:"; chkInv "Invert"
  Gain_DQNc_Mat3 : MATLAB Function  Commented=on  TreatAsAtomicUnit=on  SystemSampleTime=Ts  mask{Rabc=SYS.C, HRM=N, chkInv=off}
      mask prompts: Rabc "Line matrix [3x3]:"; HRM "Harmonic order:"; chkInv "Invert"
  Gain_DQNc_Mat4 : MATLAB Function  TreatAsAtomicUnit=on  SystemSampleTime=Ts  mask{Rabc=SYS.B, HRM=N, chkInv=off}
      mask prompts: Rabc "Line matrix [3x3]:"; HRM "Harmonic order:"; chkInv "Invert"
  Gain_DQNc_Mat5 : MATLAB Function  Commented=on  TreatAsAtomicUnit=on  SystemSampleTime=Ts  mask{Rabc=SYS.A, HRM=N, chkInv=off}
      mask prompts: Rabc "Line matrix [3x3]:"; HRM "Harmonic order:"; chkInv "Invert"
  Gain_DQNc_Mat6 : MATLAB Function  Commented=on  TreatAsAtomicUnit=on  SystemSampleTime=Ts  mask{Rabc=SYS.B, HRM=N, chkInv=off}
      mask prompts: Rabc "Line matrix [3x3]:"; HRM "Harmonic order:"; chkInv "Invert"
  Grid : Scope  NumInputPorts=4
  Ground : spsGroundLib/Ground  LConnTagsString=a
  Ihistory_Flux : Subsystem  Commented=on  AncestorBlock=DQN_Machines/DQN_Mac_V1/Ihistory_Flux
  Int_DQNc_Mat1 : MATLAB Function  Commented=on  TreatAsAtomicUnit=on  mask{N=N, dt=Ts_dqn, w=Ws, InitInt=SYS.x0, swFeed=off, R=-SYS.A, iL=eye(size(SYS.A,1))}
      mask prompts: N "Order number:"; dt "Time step (s):"; w "Angular frequency (1/rad):"; InitInt "Initial conditions DC [3x1]:"; swFeed "Enable feedback"; R "Feedback parameter (Kr {abc}):"; iL "Feedback parameter (Ki {abc}):"
  Int_DQNc_Mat6 : MATLAB Function  TreatAsAtomicUnit=on  mask{N=N, dt=Ts_dqn, w=Ws, InitInt=SYS.x0, swFeed=off, R=-SYS.A, iL=eye(size(SYS.A,1))}
      mask prompts: N "Order number:"; dt "Time step (s):"; w "Angular frequency (1/rad):"; InitInt "Initial conditions DC [3x1]:"; swFeed "Enable feedback"; R "Feedback parameter (Kr {abc}):"; iL "Feedback parameter (Ki {abc}):"
  Load Flow Bus : spsLoadFlowBusLib/Load Flow Bus  LConnTagsString=a  Phases=single  Connectors=on one side  ID=B22  Vbase=24e3  Vref=1  Vangle=0  VLF=1  VLFb=1  VLFc=1  angleLF=24.43  angleLFb=0  angleLFc=0
      settings: AttributesFormatString=%<ID>\n%<Vbase>V\n%<VLF>pu\n%<angleLF>deg.
  Load Flow Bus1 : spsLoadFlowBusLib/Load Flow Bus  LConnTagsString=a  Phases=single  Connectors=on one side  ID=BSRC  Vbase=24e3  Vref=1  Vangle=0  VLF=1  VLFb=1  VLFc=1  angleLF=0  angleLFb=0  angleLFc=0
      settings: AttributesFormatString=%<ID>\n%<Vbase>V\n%<VLF>pu\n%<angleLF>deg.
  MATLAB Function1 : MATLAB Function  Commented=on  TreatAsAtomicUnit=on  mask{N=N}
      mask prompts: N "Harmonic order:"
  MATLAB Function2 : MATLAB Function  TreatAsAtomicUnit=on  mask{N=N}
      mask prompts: N "Harmonic order:"
  MATLAB Function3 : MATLAB Function  TreatAsAtomicUnit=on  mask{N=N}
      mask prompts: N "Harmonic order:"
  MATLAB Function4 : MATLAB Function  Commented=on  TreatAsAtomicUnit=on  mask{N=N}
      mask prompts: N "Harmonic order:"
  Mac_EMT : spsSynchronousMachinepuStandardLib/Synchronous Machine pu Standard  PresetModel=No  MechanicalLoad=Mechanical power Pm  ShowDetailedParameters=on  RotorType=Round  Units=per unit standard parameters  MeasurementBus=off  NominalParameters="[ 555e6  24e3   60 ]"  Reactances1=[1.81, 0.3, 0.23, 1.76, 0.65, 0.25, 0.15]  Reactances2="[ 1.305, 0.296, 0.252, 0.474,  0.243,  0.18 ]"  dAxisTimeConstants=Short-circuit  qAxisTimeConstants=Short-circuit  TimeConstants1="[ 4.4849  0.0681  0.1  ]"  TimeConstants2=[8, 0.03, 1, 0.07]  TimeConstants3="[  4.49  0.0681  0.0513  ]"  TimeConstants4=[ 8.0, 0.03, 0.3371, 0.0295 ]  TimeConstants5=[ 1.01, 0.053, 0.1 ]  TimeConstants6=[ 1.3201, 0.023, 1.0, 0.07 ]  TimeConstants7="[  1.01  0.053  0.051266  ]"  TimeConstants8=[ 1.3201, 0.0231, 0.3371, 0.0295 ]  StatorResistance=3.10E-03  Mechanical="[ 0.8788  0 1 ]"  PolePairs=1  InitialConditions=[0 41.3296 0.910581 0.910581 0.910581 78.0886 -41.9114 198.089 1.03147]  SetSaturation=off  Saturation=[0.6404,0.7127,0.8441,0.9214,0.9956,1.082,1.19,1.316,1.457;0.7,0.7698,0.8872,0.9466,0.9969,1.046,1.1,1.151,1.201]  LoadFlowParameters=[1 0 0 0 0]  TsPowergui=0  TsBlock=Ts  IterativeModel=Trapezoidal non iterative  IterativeDiscreteModel=Trapezoidal robust  BusType=PV  Pref=299500000  Qref=-222000000  Qmin=-Inf  Qmax=Inf  PLF=0  QLF=0
  MatMux1 : Subsystem  mask{nrInp=2}
      mask prompts: nrInp "Number of inputs [{C}]"
      mask init:
      | %blocks = find_system(gcb,'LookUnderMasks','on','FollowLinks','on')
      | %set_param(gcb, 'MaskSelfModifiable', 'on');
      | 
      | % if(SSM == [])
      | %     Simulink.SubSystem.deleteContents(gcb);
      | % else
      | 
      | if(isempty(nrInp))
      |     Simulink.SubSystem.deleteContents(gcb);
      | else
      | 
      |     nrOut = 1;
      | 
      | 
      | PortHandles = get_param(gcb,'PortHandles');
      | lenInp = length(PortHandles.Inport);
      | lenOut = length(PortHandles.Inport);
      | 
      | if(nrInp ~= lenInp)
      |     %disp('ENTERED')
      |     Simulink.SubSystem.deleteContents(gcb);
      | %     add_block('simulink/Continuous/State-Space', [gcb,'/ss_block'], 'A','SS.A', 'B','SS.B', 'C','SS.C', 'D','SS.D', 'X0','X0')
      | %     set_param([gcb,'/ss_block'],'position' , [350,100,450,150])
      | 
      | 
      | 
      |         add_block('simulink/Math Operations/Matrix Concatenate',[gcb,'/Mux'], 'NumInputs',num2str(nrInp), 'ConcatenateDimension',num2str(2));
      |         set_param([gcb,'/Mux'],'position' , [200,100,250,100+nrInp*50])
      |         
      | %         add_block('built-in/Demux',[gcb,'/Demux'], 'Outputs',num2str(nrOut));
      | %         set_param([gcb,'/Demux'],'position' , [500,100,550,100+nrOut*50])
      | 
      | 
      |         for i = 1 : nrInp
      |             add_block('built-in/Inport',[gcb,strcat('/In',num2str(i))]);
      |             set_param([gcb,strcat('/In',num2str(i))],'position' , [50,65+i*50,90,85+i*50]);
      |             add_line(gcb,strcat('In',num2str(i),'/1'),strcat('Mux/',num2str(i)),'autorouting','on');
      |         end
      | 
      |         for i = 1 : nrOut
      |             add_block('built-in/Outport',[gcb,strcat('/Out',num2str(i))]);
      |             set_param([gcb,strcat('/Out',num2str(i))],'position' , [750,65+i*50,790,85+i*50]);
      |             add_line(gcb,strcat('Mux/',num2str(i)), strcat('Out',num2str(i),'/1'),'autorouting','on');
      |         end
      | 
      | 
      | %     add_line(gcb, 'Mux/1', 'ss_block/1')
      | %     add_line(gcb, 'ss_block/1', 'Demux/1')
      | 
      | end
      | 
      | end
      mask Display: disp(['{\color{red}\bf\fontsize{12}} [\{C\}]',newline,' MUX'], 'texmode','on');
  Multimeter : spsMultimeterLib/Multimeter  L=6  sel=[1 2 3]  yselected={}  Gain=[1 1 1]  OutputType=Complex  PlotAtSimulationStop=off  PhasorSimulation=off
  Multimeter1 : spsMultimeterLib/Multimeter  L=6  sel=1  yselected={}  Gain=0  OutputType=Complex  PlotAtSimulationStop=off  PhasorSimulation=off
  Mux{,1..3} (4 alike) : Mux  Inputs=2
  Mux4 : Mux  Inputs=3
  Mux5 : Mux  Inputs=3
  Mux6 : Mux  Commented=on  Inputs=2
  Mux7 : Mux  Commented=on  Inputs=3
  Mux8 : Mux  Commented=on  Inputs=3
  Mux9 : Mux  Commented=on  Inputs=2
  ParallelRLC22 : spsThreePhaseParallelRLCBranchLib/Three-Phase Parallel RLC Branch  LConnTagsString=A|B|C  RConnTagsString=A|B|C  BranchType=RC  Resistance=rlc(4,4)  Inductance=1e-3  Capacitance=rlc(4,6)*1e-6  Measurements=Branch voltages
  RL_src : spsThreePhaseSeriesRLCBranchLib/Three-Phase Series RLC Branch  LConnTagsString=A|B|C  RConnTagsString=A|B|C  BranchType=RL  Resistance=rlc(1,4)  Inductance=rlc(1,5)*1e-3  Capacitance=1/(0.55*0.080*(500e3^2/100e6))/(2*pi*60)  Measurements=Branch voltages
  SS_DQNc_Mat_Dicrete : DQN_Lib/SS_DQNc_Mat_Dicrete  Commented=on  A=SYS.A  B=SYS.B  C=SYS.C  D=SYS.D  InitVec=SYS.x0  dt=Ts  N=N  Ws=Ws
      settings: LibrarySourceBlock=|
      | spsSynchronousMachineModel/Discrete robust/State Space Model/Discretize
      | BE or Tustin
  SS_DelayPrediction : DQN_Lib/SS_DelayPrediction  N=N  Ts=Ts  x0=SYS.x0
  SS_DelayPrediction1 : DQN_Lib/SS_DelayPrediction  Commented=on  N=N  Ts=Ts  x0=SYS.x0
  Selector1 : Selector  Commented=on  InputPortWidth=3  IndexOptions=Index vector (dialog)  Indices=[1 2]  OutputSizes=1
  Selector2 : Selector  InputPortWidth=3  IndexOptions=Index vector (dialog)  Indices=[1 2]  OutputSizes=1
  Selector3 : Selector  InputPortWidth=3  IndexOptions=Index vector (dialog)  Indices=[1 2]  OutputSizes=1
  Selector4 : Selector  Commented=on  InputPortWidth=3  IndexOptions=Index vector (dialog)  Indices=[1 2]  OutputSizes=1
  State-Space : StateSpace  Commented=on  A=SYS.A1  B=SYS.B1  C=SYS.C1  D=SYS.D  InitialCondition=InitVec
  Steam Turbine and Governor : spsSteamTurbineandGovernorLib/Steam Turbine and Governor  gentype=Tandem-compound (multi-mass)  reg1="[ 1  0.05    0 ]"  reg2="[ 0.001  0.15 ]"  reg3="[ -0.1  0.1  0  4.496]"  N=3600  turb1="[ 0  10   3.3   0.5   ]"  turb2="[ 0.5   0.5   0  0 ]"  HA="[  1.5498   0.24894  0  0 ]"  KA="[  83.47  42.702  0  0 ]"  DA="[  0.3104  0.05  0  0 ]*8"  ini1=250.35/555  ini2=[0.54221 41.33]
  Steam Turbine and Governor1 : Subsystem  DialogController=POWERSYS.PowerSysDialog  mask(Steam Turbine and Governor){gentype=Tandem-compound (multi-mass), reg1=[ 1  0.05    0 ], reg2=[ 0.001  0.15 ], reg3=[ -0.1  0.1  0  4.496], N=3600, turb1=[ 0  10   3.3   0.5   ], turb2=[ 0.5   0.5   0  0 ], HA=[  1.5498   0.24894  0  0 ], KA=[  83.47  42.702  0  0 ], DA=[  0.3104  0.05  0  0 ]*8, ini1=250.35/555, ini2=[0.54221 41.33]}
      mask prompts: gentype "Generator type"; reg1 "Regulator gain, perm. droop, dead zone [ Kp  Rp(pu)  Dz(pu) ]:"; reg2 "Speed relay and servo-motor time constants [ Tsr  Tsm ] (s):"; reg3 "Gate opening limits [ vgmin,vgmax (pu/s)  gmin,gmax (pu)]:"; N "Nominal speed of synchronous machine (rpm)"; turb1 "Steam turbine time constants [ T2  T3  T4  T5 ] (s):"; turb2 "Turbine torque fractions [ F2  F3  F4  F5 ]:"; HA "Coeff. of inertia [ H2  H3  H4  H5 ] (s):"; KA "Stiffness coeff. [ K12  K23  K34  K45 ] (pu/rad):"; DA "Damping factors [ D2  D3  D4  D5 ] (pu T/pu dw):"; ini1 "Initial power Pm0 (pu):"; ini2 "Initial power and generator rotor angle [ Pm0 (pu)  th0(deg) ]:"
      mask help:
      | Implements a complete tandem-compound steam prime mover system, including
      | speed regulator, steam turbine and a shaft with up to 4 masses. The genererator's
      | mass is labelled mass #1 and is not included here. The shaft mass closest to the
      | generator is #2, the farthest is #5. If a mass is not to be included, set it's inertia H to
      | zero. The damping factor and rigidity coefficients corresponding to omitted masses
      | are not considered and can be left as is. When masses are omitted, the remaining
      | system is "compressed" towards the generator i.e. if only 2 masses are used, it will
      | be masses #2 and #3. The input data for the masses considered is shifted accordingly.
      mask init:
      | block = gcb;
      | [Ts, WantBlockChoice, q0,FA,Ha,Ka,Da,dtha,t,errorFlag,ctrl1,sel,massNumber] = powericon('SteamTurbineInit',gcb,gentype,reg1,reg2,reg3,turb1,turb2,HA,KA,DA,ini1,ini2);
      | powericon('SetInternalModels','set',block,WantBlockChoice);
      settings: OpenFcn=sps_rtmsupport('OpenFcn',gcbh)
      settings: LibrarySourceBlock=|
      | spsSteamTurbineandGovernorLib/Steam Turbine
      | and Governor
      mask Help: helpview(psbhelp);
      mask TypeOptions gentype: Tandem-compound (single mass) | Tandem-compound (multi-mass)
      mask Callback gentype: powericon('psbcallbacks',gcbh,'SteamTurbine');
      mask Display: plot([0 0],[t t])
  Step1 : Step  Time=5  Before=0.54221  After=0.54221  SampleTime=0
  Step2 : Step  Time=7  Before=1.0315  After=10  SampleTime=0
  Subsystem : Subsystem
  Terminator : Terminator
  To Workspace : ToWorkspace  Commented=on  VariableName=InitVec  SampleTime=Ts
      settings: MaxDataPoints=1
  Turbine : Scope  NumInputPorts=3
  V2kV : Gain  Gain=1/1000
  XY1 : Scope  Commented=on  NumInputPorts=2
  XY2 : Scope  NumInputPorts=3
  XY3 : Scope  NumInputPorts=2
  abc to dq1 : spsabctodq0Lib/abc to dq0  Commented=on  Alignment=90 degrees behind phase A axis
  abc to dq2 : spsabctodq0Lib/abc to dq0  Alignment=90 degrees behind phase A axis
  abc to dq3 : spsabctodq0Lib/abc to dq0  Alignment=90 degrees behind phase A axis
  abc to dq4 : spsabctodq0Lib/abc to dq0  Commented=on  Alignment=90 degrees behind phase A axis
  last column of D : Selector  Commented=on  NumberOfDimensions=2  InputPortWidth=3  IndexOptions=Index vector (dialog),Index vector (dialog)  Indices=[1:SMRD.nState],3  OutputSizes=1,1
  powergui : spspowerguiLib/powergui  Priority=2  SimulationMode=Discrete  SampleTime=Ts  frequency=60  Iterations=50  frequencyindice=60  Pbase=100e6  ErrMax=0.0001  UnitsV=kV  UnitsW=MW  buscounter=0  FunctionMessages=off  echomessages=off  EnableUseOfTLC=off  CurrentSourceSwitches=off  DisableSnubberDevices=off  DisableRonSwitches=off  DisableVfSwitches=off  DisplayEquations=off  AutomaticDiscreteSolvers=off  SolverType=Tustin/Backward Euler (TBE)  Interpol=off  ExternalGateDelay=off  methode=off  Ts=0  x0status=blocks  SPID=on  SwTol=0  HookPort=off  NonlinearTolerance=1e-4  nMaxIteration=100  ContinueOnMaxIteration=off  RestoreLinks=warning  ResistiveCurrentMeasurement=off  Frange=logspace(0,3,50)  Ylog=off  Xlog=off  ShowGrid=off  save=off  variable=ZData  structure=0  ZoomFFT=on  StartTime=0.0  cycles=2  DisplayStyle=off  fundamental=60  FreqAxis=off  MaxFrequency=1000  frequencyindicesteady=1  RmsSteady=1  display=off
  wires:
  [Vabc_B500] -> Grid/1  "Vabc_B500 (pu)"
  [Iabc_B222] -> Grid/2  "Iabc_B22 (A)"
  Multimeter/1 -> V2kV/1  "V series capacitors (pu)"
  V2kV/1 -> Grid/3  "V series capacitors (kV)"
  Multimeter1/1 -> Grid/4  "I_Fault (A)"
  Steam Turbine and Governor/4 -> [Pm], Turbine/3, Mac_EMT/1
  Steam Turbine and Governor/3 -> Terminator/1
  [Pref] -> Steam Turbine and Governor/2
  Bus Selector1/2 -> Steam Turbine and Governor/3  "<Rotor speed  wm  (pu)>"
  Subsystem/2(T_23) -> Turbine/2  "T2 (Gen-LP)  T3(LP-HP)  [pu]"
  Bus Selector1/3 -> Subsystem/1(In1)  "<Rotor speed deviation  dw (pu)>"
  Steam Turbine and Governor/1 -> Subsystem/2(In2)
  Mac_EMT/1 -> Bus Selector2/1, Bus Selector1/1
  Subsystem/1(dw_123) -> Turbine/1  "dw1(Gen)  dw2(LP)   dw3(HP) [pu]"
  Bus Selector1/1 -> Steam Turbine and Governor/4  "<Rotor angle deviation  d_theta (rad)>"
  Constant5/1 -> Steam Turbine and Governor/1
  Steam Turbine and Governor/2 -> Subsystem/3(In3)
  DQN_Mac1_V1/1(I_C) -> [Igc_C], DQn->ABC/1(Xdcpnz_c)  "[N+1,18 (6+6+6)]"
  Constant2/1 -> [VSRC_C]
  Int_DQNc_Mat6/1(Zpnz) -> SS_DelayPrediction/1
  SS_DelayPrediction/1 -> Gain_DQNc_Mat1/1(Xpnz), Gain_DQNc_Mat2/1(Xpnz)  "dw"
  Gain_DQNc_Mat4/1(Ypnz) -> Add1/1
  Add1/1 -> Int_DQNc_Mat6/1(Xpnz)
  Gain_DQNc_Mat2/1(Ypnz) -> Add1/2
  MATLAB Function2/1(Vs_c) -> MatMux1/2(In2)
  Demux6/2 -> Mux1/2  "Mac_SS_b"
  Demux7/2 -> Mux1/1  "Mac_EMT_b"
  DQn->ABC/1(Xabc) -> Demux6/1  "Mac_EMT"
  Demux7/1 -> Mux3/1  "Mac_EMT_a"
  Mux1/1 -> XY2/2
  Mux3/1 -> XY2/1
  Demux7/3 -> Mux2/1  "Mac_EMT_c"
  Demux6/3 -> Mux2/2  "Mac_SS_c"
  Demux6/1 -> Mux3/2  "Mac_SS_a"
  [Iabc_B222] -> Demux7/1  "Iabc_B22 (A)"
  Mux2/1 -> XY2/3
  From12/1 -> abc to dq1/2  "theta"
  abc to dq1/1 -> Selector1/1  "vq,vd"
  Selector1/1 -> MATLAB Function1/1(Vdq_vec)
  From18/1 -> abc to dq1/1  "v"
  Clock/1 -> Gain12/1
  Gain12/1 -> [theta0]
  [Pref] -> Steam Turbine and Governor1/2(Pref)
  Constant1/1 -> Steam Turbine and Governor1/1(wref)
  Step2/1 -> Mac_EMT/2, [Vf]
  [theta0] -> DQn->ABC/2(tho)  "theta"
  [Iabc_B222] -> Mux/1  "Iabc_B22 (A)"
  Mux4/1 -> XY3/1
  Mux5/1 -> XY3/2
  [Vabc_B22] -> Mux4/1  "Vabc_EMT"
  [Iabc_B500] -> Gain1/1  "Iabc_B22 (A)"
  Demux/2 -> Mux5/2  "Iabc_SS"
  Demux/1 -> Mux4/2  "Vabc_SS"
  Gain1/1 -> Mux5/1  "Iabc_EMT"
  Demux_DQNc_Mat2/1 -> DQN_Mac1_V1/1(Vs_C), DQn->ABC1/1(Xdcpnz_c)  "[N+1,18 (6+6+6)]"
  Step1/1 -> [Pref]
  [theta0] -> DQn->ABC1/2(tho)  "theta"
  [theta0] -> DQn->ABC2/2(tho)  "theta"
  Demux_DQNc_Mat2/2 -> DQn->ABC2/1(Xdcpnz_c)  "[N+1,18 (6+6+6)]"
  DQn->ABC2/1(Xabc) -> Mux5/3  "Iabc_DQN"
  DQn->ABC1/1(Xabc) -> Mux4/3  "Vabc_DQN"
  [Vabc_BSRC] -> abc to dq2/1  "v"
  [theta0] -> abc to dq2/2  "theta"
  abc to dq2/1 -> Selector2/1  "vq,vd"
  Selector2/1 -> MATLAB Function2/1(Vdq_vec)
  [Vabc_BSRC] -> Mux/2  "v"
  Mux/1 -> Discrete State-Space/1
  Discrete State-Space/1 -> Demux/1
  abc to dq3/1 -> Selector3/1  "vq,vd"
  [Vabc_B22] -> abc to dq3/1  "v"
  [theta0] -> abc to dq3/2  "theta"
  Selector3/1 -> MATLAB Function3/1(Vdq_vec)
  [Igc_C] -> MatMux1/1(In1)
  MatMux1/1(Out1) -> Gain_DQNc_Mat4/1(Xpnz)
  Gain_DQNc_Mat1/1(Ypnz) -> Demux_DQNc_Mat2/1
  DQN_Mac1_V1/2(dtheta_e) -> Steam Turbine and Governor1/4(d_theta)
  DQN_Mac1_V1/3(wm) -> Steam Turbine and Governor1/3(wm)
  [Vf] -> DQN_Mac1_V1/2(Vf)
  Steam Turbine and Governor1/1(Pm) -> DQN_Mac1_V1/3(Pm)
  Bus Selector2/1 -> Display1/1
  Constant7/1 -> Discretize BE or Tustin/3(C)
  Discretize BE or Tustin/3(Cd) -> Ihistory_Flux/5(Cd)
  Discretize BE or Tustin/1(Ad) -> Ihistory_Flux/3(Ad)
  Constant3/1 -> Discretize BE or Tustin/1(A)
  Discretize BE or Tustin/4(Dd) -> Ihistory_Flux/6(D(:,3))
  Constant6/1 -> Ihistory_Flux/2(B), Discretize BE or Tustin/2(B)
  Discretize BE or Tustin/2(Bd) -> Ihistory_Flux/4(Bd)
  From5/1 -> abc to dq4/2  "theta"
  Selector4/1 -> MATLAB Function4/1(Vdq_vec)
  From6/1 -> abc to dq4/1  "v"
  Discretize BE or Tustin/5(inv(I_Ts/2*A)) -> Ihistory_Flux/7(inv())
  abc to dq4/1 -> Selector4/1  "vq,vd"
  From24/1 -> Gain3/1  "Iabc_B22 (A)"
  From23/1 -> Mux9/1  "Vabc_EMT"
  Discrete State-Space1/1(Y) -> Demux1/1
  Gain3/1 -> Mux9/2  "Iabc_EMT"
  From20/1 -> DQn->ABC3/2(tho)  "theta"
  Mux8/1 -> XY1/2
  Gain2/1 -> Mux8/1  "Iabc_EMT"
  From27/1 -> Mux7/1  "Vabc_EMT"
  ? -> DQn->ABC4/1(Xdcpnz_c)  "[N+1,18 (6+6+6)]"
  Mux7/1 -> XY1/1
  ? -> DQn->ABC3/1(Xdcpnz_c)  "[N+1,18 (6+6+6)]"
  From22/1 -> DQn->ABC4/2(tho)  "theta"
  Mux9/1 -> To Workspace/1, Display2/1
  DQn->ABC3/1(Xabc) -> Mux7/3  "Vabc_DQN"
  DQn->ABC4/1(Xabc) -> Mux8/3  "Iabc_DQN"
  Mux6/1 -> Discrete State-Space1/1(U)
  From21/1 -> Mux6/2  "v"
  From26/1 -> Gain2/1  "Iabc_B22 (A)"
  SS_DelayPrediction1/1 -> Gain_DQNc_Mat3/1(Xpnz), Gain_DQNc_Mat5/1(Xpnz)  "dw"
  ? -> Gain_DQNc_Mat6/1(Xpnz)
  Gain_DQNc_Mat6/1(Ypnz) -> Add2/1
  Int_DQNc_Mat1/1(Zpnz) -> SS_DelayPrediction1/1  "dw"
  Demux1/2 -> Mux8/2  "Iabc_SS"
  Add2/1 -> Int_DQNc_Mat1/1(Xpnz)
  Gain_DQNc_Mat3/1(Ypnz) -> ?
  From25/1 -> Mux6/1  "Iabc_B22 (A)"
  Demux1/1 -> Mux7/2  "Vabc_SS"
  Gain_DQNc_Mat5/1(Ypnz) -> Add2/2
  connections:
  RL_src/RConn2 -- B500/RConn2
  B500/RConn1 -- RL_src/RConn1
  RL_src/RConn3 -- B500/RConn3
  B22/LConn1 -- Mac_EMT/RConn1 -- Load Flow Bus/LConn1
  ParallelRLC22/LConn1 -- B500/LConn1 -- B22/RConn1
  B22/RConn2 -- B500/LConn2 -- ParallelRLC22/LConn2
  ParallelRLC22/LConn3 -- B500/LConn3 -- B22/RConn3
  B1/LConn1 -- RL_src/LConn1
  Ground/LConn1 -- ParallelRLC22/RConn2 -- ParallelRLC22/RConn3 -- ParallelRLC22/RConn1
  RL_src/LConn2 -- B1/LConn2
  RL_src/LConn3 -- B1/LConn3
  B1/RConn1 -- Load Flow Bus1/LConn1 -- 500 kV 3333 MVA/RConn1
  B1/RConn2 -- 500 kV 3333 MVA/RConn2
  B1/RConn3 -- 500 kV 3333 MVA/RConn3
  Mac_EMT/RConn3 -- B22/LConn3
  Mac_EMT/RConn2 -- B22/LConn2
